simulink model "zoomLensWithLookupTbl"  (Simulink 6.1)
settings: Solver=ode45  StartTime=0.0  StopTime=3  RelTol=1e-3
undefined symbols (not defined in the file or in its folder): mag, reading
settings Model: LastModifiedBy=Big E
settings DebuggingCC: SolverPrmCheckMsg=warning

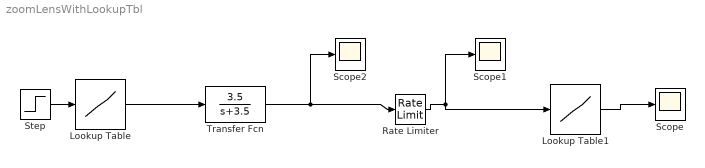
== system zoomLensWithLookupTbl ==
  Lookup Table : Lookup  DialogController=Simulink.DDGSource  InputValues=mag  OutputValues=reading  LookUpMeth=Interpolation-Use End Values
  Lookup Table1 : Lookup  DialogController=Simulink.DDGSource  InputValues=reading  OutputValues=mag  LookUpMeth=Interpolation-Use End Values
  Rate Limiter : RateLimiter  RisingSlewLimit=14130  FallingSlewLimit=-14130  SampleTimeMode=inherited
  Scope : Scope
      settings: YMin=0  YMax=750
  Scope1 : Scope
      settings: YMin=0  YMax=750
  Scope2 : Scope
      settings: YMin=0  YMax=750  SaveName=ScopeData2
  Step : Step  After=20  SampleTime=0
  Transfer Fcn : TransferFcn  Numerator=[3.5]  Denominator=[1 3.5]
  wires:
  Transfer Fcn/1 -> Rate Limiter/1, Scope2/1
  Rate Limiter/1 -> Scope1/1, Lookup Table1/1
  Lookup Table/1 -> Transfer Fcn/1
  Step/1 -> Lookup Table/1
  Lookup Table1/1 -> Scope/1
